simulink library "measurement_tools"  (Simulink 8.6)
settings: Solver=ode45  SolverMode=SingleTasking  StartTime=0.0  StopTime=10.0  RelTol=1e-3
values from neighbouring files (symbols this model uses):
  D = 'STP4'    [digital_communications_gui.m]
undefined symbols (not defined in the file or in its folder): DiscIntNeverNeededParam, get
libraries: dspsigops x3, dspsnks4 x2, dspvision x2, simulink_extras x1, dspswit3 x1, dspobslib x1, simulink x1
settings Model: MAModelExclusionFileProxy=C:\Users\user\Desktop\HAW\Digital Communication Systems\labs\Matlab\measurement_tools_exclusions.xml  Creator=Schoenen  LastModifiedBy=user

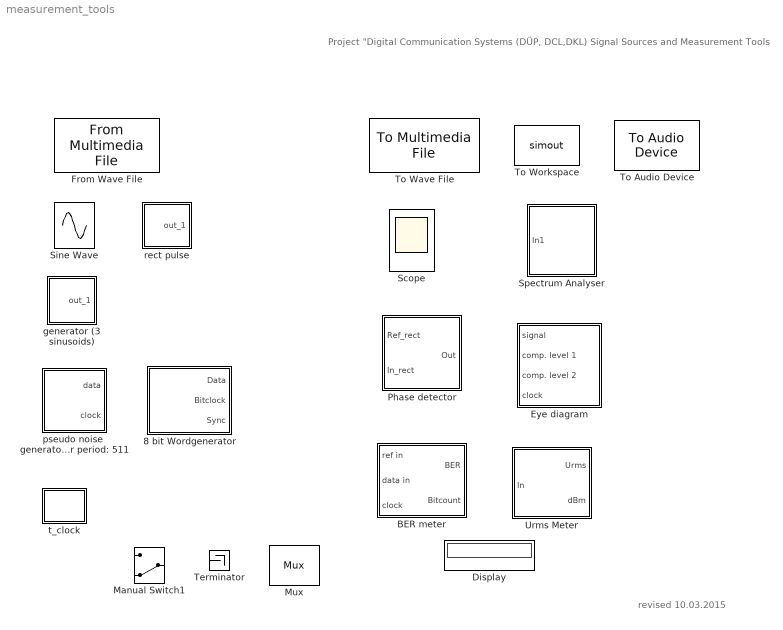
== system measurement_tools ==
  note: revised 10.03.2015
  note: Project "Digital Communication Systems (DÜP, DCL,DKL)
      | Signal Sources and Measurement Tools
  8 bit Wordgenerator : Subsystem  mask{word=[0 0 0 0 0 0 0 0], bt=1}
      mask prompts: word "8 Bit Word (enter vector)"; bt "Bitclock [Hz]"
      mask help: 8 Bit Wordgenerator
  BER meter : Subsystem
  Display : Display
      settings: Format=short_e
  Eye diagram : Subsystem  mask{Tsymb=1, Tfss=2/64e5, ns=4, ndisplay=1, ymin=1, ymax=1}
      mask prompts: Tsymb "symbol period [s]:"; Tfss "simulation step size [s]:"; ns "symbols per eye diagram (min. 4xndisplay):"; ndisplay "display time scale [ndisplay=number of symbols]:"
      mask init:
      | SampPerSymb = round(Tsymb/Tfss);
      | nsymb=ndisplay*ceil(ns/ndisplay);
  From Wave File : dspvision/From Multimedia File  inputFilename=audio_in_8kHz.wav  loop=on  numPlays=1  outputStreams=Audio only  videoDataType=single  audioDataType=double  inheritSampleTime=on  userDefinedSampleTime=1/30  noAudioOutput=off  isIntensityVideo=off  fourcc=RGB  colorVideoFormat=Separate color signals  outputEOF=off  dataOrg=Column-major  audioFrameSize=1  computeAudioFrameSize=off  outSamplingMode=Sample based
  Manual Switch1 : ManualSwitch  CurrentSetting=0
  Mux : Mux  Inputs=2
  Phase detector : Subsystem
  Scope : Scope
  Sine Wave : Sin  Amplitude=0  SampleTime=0
  Spectrum Analyser : Subsystem  mask{st=1}
      mask prompts: st "sample time [s]"
      mask help: Spectrum-Analyser
  Terminator : Terminator
  To Audio Device : dspsnks4/To Audio Device  deviceName=Default  inheritSampleRate=on  sampleRate=44100  deviceDatatype=Determine from input data type  autoBufferSize=on  bufferSize=4096  queueDuration=0.2  defaultOutputChannelMapping=on  outputChannelMapping=1:2  outputNumUnderrunSamples=off
  To Wave File : dspvision/To Multimedia File  outputFilename=audio_out.wav  streamSelection=Audio only  videoCompressor=None (uncompressed)  audioCompressor=None (uncompressed)  imagePorts=Separate color signals  fileType=WAV  audioDatatype=16-bit integer  fourcc=RGB  videoQuality=75  mj2000CompFactor=10
  To Workspace : ToWorkspace  VariableName=simout  SaveFormat=Structure  SampleTime=-1
  Urms Meter : Subsystem  mask{T=1}
      mask prompts: T "integration time [s]"
  generator (3 sinusoids) : Subsystem  mask(3_Tongenerator){}
      mask help: 3-Tongenerator
      mask init:
      | a1=@1(1); a2=@2(1); a3=@3(1); f1=@1(2); f2=@2(2); f3=@3(2); p1=@1(3); p2=@2(3); p3=@3(3);
      mask Help: Der Generator erzeugt eine Summe aus drei \nSinusschwingungen unterschiedlicher Amplitude \nund Phasenlage. Die Schwingungsparameter \nwerden jeweils als Vektor in der Form \n[Amplitude Frequenz Phase] eingegeben.
  pseudo noise  generator period: 511 : Subsystem  AncestorBlock=|  mask(pseudo noise generator){Tsymb=1, pol=unipolar, Tfss=2/64e5}
      | measuring_tools/pseudo noise
      |  generator
      | period: 511
      mask prompts: Tsymb "symbol period [s]"; pol "signal"; Tfss "simulation step size [s]"
      mask help: generates a periodical pseudo noise sequence (period Tp=511 Tbit)
      mask TypeOptions pol: bipolar | unipolar
  rect pulse : Subsystem  mask(Einheitsimpuls){breite=1, start=1}
      mask prompts: breite "width [s]"; start "start time [s]"
      mask help: Einheitsimpuls
      mask Help: Einheitsimpuls mit der Fläche 1
      mask Display: plot([0 0 0 0 1 0 0 0 0 0 0 0 0 0 0 0 0 0 0 0 ])
  t_clock : Subsystem
      mask init:
      | block_symbol=[0 1 0 0 0 0 0 0 0  1 0 0 0 0 0 0 01];
      mask Display: plot(block_symbol);

== system measurement_tools/8 bit Wordgenerator ==
  Clock-Generator : Subsystem  mask{bt=64e3}
      mask prompts: bt "Bitclock"
      mask help: Clock-Generator
  Parallel-Serial : Subsystem
  Word : Constant  Value=word
  Data : Outport
  Bitclock : Outport  Port=2
  Sync : Outport  Port=3
  wires:
  Parallel-Serial/1(Data_out) -> Data/1
  Word/1 -> Parallel-Serial/1(Data_in)
  Clock-Generator/2(Wordclock) -> Sync/1, Parallel-Serial/2(Preset)
  Clock-Generator/1(Bitclock) -> Bitclock/1, Parallel-Serial/3(Clock)

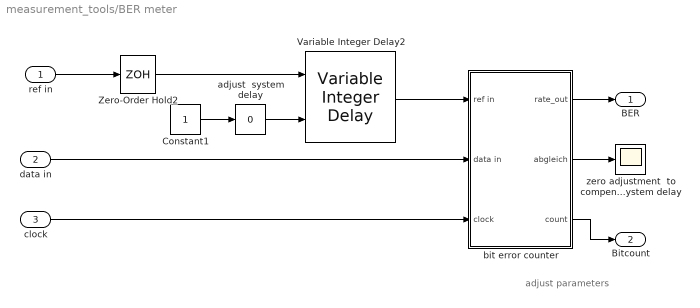
== system measurement_tools/BER meter ==
  note: adjust parameters
  ref in : Inport
  data in : Inport  Port=2
  clock : Inport  Port=3
  " bit error counter" : Subsystem  AncestorBlock=measuring_tools/discrete bit error counter  mask{Tbit=1, M=1}
      mask prompts: Tbit "bit period [s]"; M "measuring over number of bits:"
  Constant1 : Constant
  Variable Integer Delay2 : dspobslib/Variable Integer Delay  dmax=100  InputProcessing=Inherited (this choice will be removed - see release notes)  ic=0  noDFT=off
  Zero-Order Hold2 : ZeroOrderHold  SampleTime=2/64e5
  adjust  system delay : simulink/Math Operations/Slider Gain  low=0  gain=0  high=100
  zero adjustment  to compensate  system delay : Scope
  BER : Outport
  Bitcount : Outport  Port=2
  wires:
  " bit error counter"/3(count) -> Bitcount/1
  adjust  system delay/1 -> Variable Integer Delay2/2
  Constant1/1 -> adjust  system delay/1
  Zero-Order Hold2/1 -> Variable Integer Delay2/1
  Variable Integer Delay2/1 -> " bit error counter"/1(ref in)
  ref in/1 -> Zero-Order Hold2/1
  data in/1 -> " bit error counter"/2(data in)
  clock/1 -> " bit error counter"/3(clock)
  " bit error counter"/1(rate_out) -> BER/1
  " bit error counter"/2(abgleich) -> zero adjustment  to compensate  system delay/1

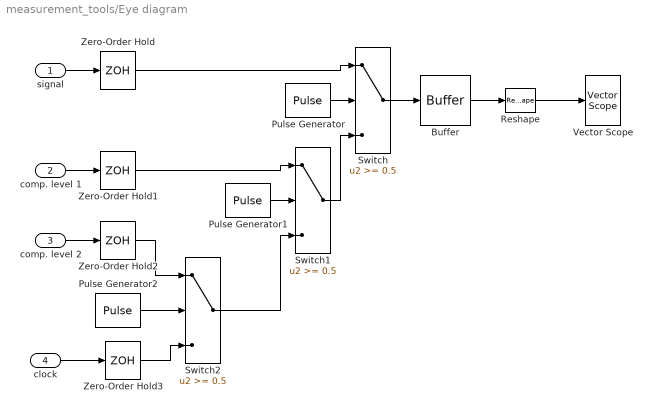
== system measurement_tools/Eye diagram ==
  signal : Inport
  comp. level 1 : Inport  Port=2
  comp. level 2 : Inport  Port=3
  clock : Inport  Port=4
  Buffer : Buffer  RequirementInfo="{}  %GIDa_20dddd1b_447a_4159_b5a4_549dd01b317e"  N=nsymb*SampPerSymb
  Pulse Generator : DiscretePulseGenerator  Period=nsymb*SampPerSymb  PulseWidth=(nsymb-3*ndisplay)*SampPerSymb  PhaseDelay=3*ndisplay*SampPerSymb  SampleTime=Tfss
  Pulse Generator1 : DiscretePulseGenerator  Period=nsymb*SampPerSymb  PulseWidth=ndisplay*SampPerSymb  SampleTime=Tfss
  Pulse Generator2 : DiscretePulseGenerator  Period=nsymb*SampPerSymb  PulseWidth=ndisplay*SampPerSymb  PhaseDelay=ndisplay*SampPerSymb  SampleTime=Tfss
  Reshape : Reshape  OutputDimensionality=Customize  OutputDimensions=[ndisplay*SampPerSymb,nsymb/ndisplay]
  Switch : Switch  Threshold=0.5  SaturateOnIntegerOverflow=on
  Switch1 : Switch  Threshold=0.5  SaturateOnIntegerOverflow=on
  Switch2 : Switch  Threshold=0.5  SaturateOnIntegerOverflow=on
  Vector Scope : dspsnks4/Vector Scope  ScopeProperties=off  Domain=Time  HorizSpan=1  DisplayProperties=off  AxisGrid=on  Memory=on  FrameNumber=on  AxisLegend=off  AxisZoom=off  OpenScopeAtSimStart=on  OpenScopeImmediately=off  FigPos=get(0,'defaultfigureposition')  AxisProperties=on  XUnits=Hertz  XRange=[0...Fs/2]  InheritXIncr=on  XIncr=1  XLabel=Time  XLimit=Auto  XMin=0  XMax=1  XStart=0  YUnits=dB  YLabel=Amplitude  LineProperties=off  LineColors=[1 0 0]|[0 1 0]|[0 0 1]  XAxisParamsVer=6.8
      settings: YMin=ymin  YMax=ymax
  Zero-Order Hold{,1..3} (4 alike) : ZeroOrderHold  SampleTime=Tfss
  wires:
  Pulse Generator2/1 -> Switch2/2
  Switch2/1 -> Switch1/3
  Zero-Order Hold3/1 -> Switch2/3
  clock/1 -> Zero-Order Hold3/1
  Zero-Order Hold2/1 -> Switch2/1
  comp. level 2/1 -> Zero-Order Hold2/1
  comp. level 1/1 -> Zero-Order Hold1/1
  signal/1 -> Zero-Order Hold/1
  Switch1/1 -> Switch/3
  Pulse Generator1/1 -> Switch1/2
  Zero-Order Hold1/1 -> Switch1/1
  Pulse Generator/1 -> Switch/2
  Switch/1 -> Buffer/1
  Zero-Order Hold/1 -> Switch/1
  Reshape/1 -> Vector Scope/1
  Buffer/1 -> Reshape/1

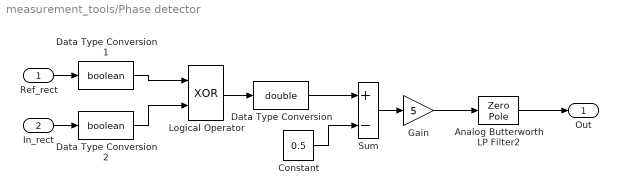
== system measurement_tools/Phase detector ==
  Ref_rect : Inport
  In_rect : Inport  Port=2
  Analog Butterworth LP Filter2 : ZeroPole  Zeros=z  Poles=p  Gain=k  mask(buttap){}
      mask help:
      | Analog Butterworth low pass filter.
      |
      | (Requires Signal Processing Toolbox)
      mask init:
      | [z,p,k]=buttap(@2); z=@1*z; p=@1*p; k=real(prod(-p)); [num,den]=zp2tf(z,p,k); w=logspace(log10(@1/10),log10(10*@1),20); h=freqs(num,den,w);
      mask Help: Butterworth low pass filter using MATLAB's butter command.
      mask Display: plot(20*log10(w),20*log10(abs(h)))
  Constant : Constant  Value=0.5
  Data Type Conversion : DataTypeConversion  OutDataTypeStr=double  SaturateOnIntegerOverflow=on  RndMeth=Zero
  Data Type Conversion1 : DataTypeConversion  OutDataTypeStr=boolean  SaturateOnIntegerOverflow=on  RndMeth=Zero
  Data Type Conversion2 : DataTypeConversion  OutDataTypeStr=boolean  SaturateOnIntegerOverflow=on  RndMeth=Zero
  Gain : Gain  Gain=5  SaturateOnIntegerOverflow=on  OutDataTypeStr=Inherit: Same as input  ParamDataTypeStr=Inherit: Same as input
  Logical Operator : Logic  Operator=XOR
  Sum : Sum  Inputs=+-  SaturateOnIntegerOverflow=on
  Out : Outport
  wires:
  In_rect/1 -> Data Type Conversion2/1
  Gain/1 -> Analog Butterworth LP Filter2/1
  Ref_rect/1 -> Data Type Conversion1/1
  Sum/1 -> Gain/1
  Constant/1 -> Sum/2
  Data Type Conversion/1 -> Sum/1
  Logical Operator/1 -> Data Type Conversion/1
  Data Type Conversion2/1 -> Logical Operator/2
  Data Type Conversion1/1 -> Logical Operator/1
  Analog Butterworth LP Filter2/1 -> Out/1

== system measurement_tools/Spectrum Analyser ==
  In1 : Inport
  Spectrum Scope : SpectrumAnalyzer
  Zero-Order Hold : ZeroOrderHold  SampleTime=st
  wires:
  In1/1 -> Zero-Order Hold/1
  Zero-Order Hold/1 -> Spectrum Scope/1

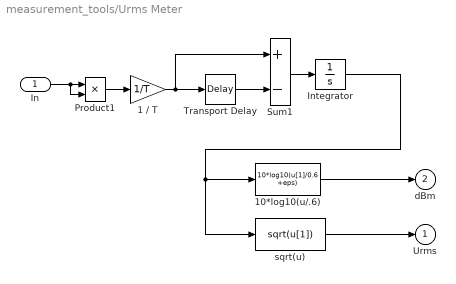
== system measurement_tools/Urms Meter ==
  In : Inport
  1 / T : Gain  Gain=1/T  SaturateOnIntegerOverflow=on  OutDataTypeStr=Inherit: Same as input  ParamDataTypeStr=Inherit: Same as input
  10*log10(u/.6) : Fcn  Expr=10*log10(u[1]/0.6 +eps)
  Integrator : Integrator
  Product1 : Product  SaturateOnIntegerOverflow=on  InputSameDT=on  OutDataTypeStr=Inherit: Same as first input
  Sum1 : Sum  Inputs=+-  SaturateOnIntegerOverflow=on  InputSameDT=on  OutDataTypeStr=Inherit: Same as first input
  Transport Delay : TransportDelay  DelayTime=T  BufferSize=1024*8
  sqrt(u) : Fcn  Expr=sqrt(u[1])
  Urms : Outport  InitialOutput=0
  dBm : Outport  Port=2  InitialOutput=0
  wires:
  sqrt(u)/1 -> Urms/1
  In/1 -> Product1/2, Product1/1
  Sum1/1 -> Integrator/1
  Transport Delay/1 -> Sum1/2
  1 / T/1 -> Sum1/1, Transport Delay/1
  Integrator/1 -> 10*log10(u/.6)/1, sqrt(u)/1
  10*log10(u/.6)/1 -> dBm/1
  Product1/1 -> 1 / T/1

== system measurement_tools/generator (3 sinusoids) ==
  Clock : Clock
  NF : Fcn  Expr=a1*sin(2*pi*f1*u+p1)
  NF1 : Fcn  Expr=a2*sin(2*pi*f2*u+p2)
  NF4 : Fcn  Expr=a3*sin(2*pi*f3*u+p3)
  Sum : Sum  Inputs=+++  SaturateOnIntegerOverflow=on  InputSameDT=on  OutDataTypeStr=Inherit: Same as first input
  out_1 : Outport
  wires:
  Sum/1 -> out_1/1
  NF/1 -> Sum/1
  NF1/1 -> Sum/2
  NF4/1 -> Sum/3
  Clock/1 -> NF1/1, NF/1, NF4/1

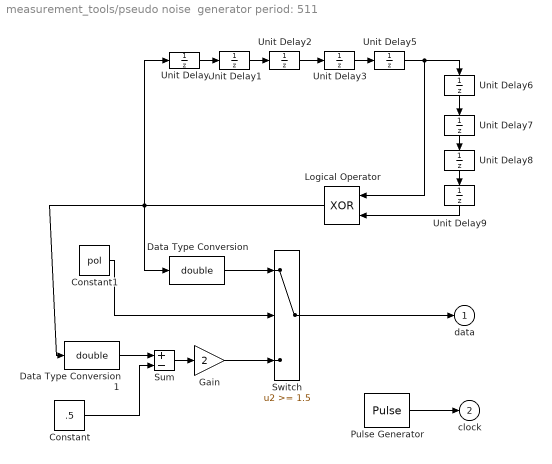
== system measurement_tools/pseudo noise  generator period: 511 ==
  Constant : Constant  Value=.5
  Constant1 : Constant  Value=pol
  Data Type Conversion : DataTypeConversion  OutDataTypeStr=double  SaturateOnIntegerOverflow=on  RndMeth=Zero
  Data Type Conversion1 : DataTypeConversion  OutDataTypeStr=double  SaturateOnIntegerOverflow=on  RndMeth=Zero
  Gain : Gain  Gain=2  SaturateOnIntegerOverflow=on  OutDataTypeStr=Inherit: Same as input  ParamDataTypeStr=Inherit: Same as input
  Logical Operator : Logic  Operator=XOR
  Pulse Generator : DiscretePulseGenerator  Period=round(Tsymb/Tfss)  SampleTime=Tfss
  Sum : Sum  Inputs=+-  SaturateOnIntegerOverflow=on  InputSameDT=on  OutDataTypeStr=Inherit: Same as first input
  Switch : Switch  Threshold=1.5  SaturateOnIntegerOverflow=on  InputSameDT=on
  Unit Delay : UnitDelay  InitialCondition=1  SampleTime=Tsymb
  Unit Delay{1..3,5..9} (8 alike) : UnitDelay  SampleTime=Tsymb
  data : Outport  InitialOutput=0
  clock : Outport  Port=2
  wires:
  Pulse Generator/1 -> clock/1
  Constant1/1 -> Switch/2
  Logical Operator/1 -> Unit Delay/1, Data Type Conversion1/1, Data Type Conversion/1
  Gain/1 -> Switch/3
  Switch/1 -> data/1
  Constant/1 -> Sum/2
  Sum/1 -> Gain/1
  Unit Delay5/1 -> Unit Delay6/1, Logical Operator/1
  Unit Delay3/1 -> Unit Delay5/1
  Unit Delay2/1 -> Unit Delay3/1
  Unit Delay9/1 -> Logical Operator/2
  Unit Delay8/1 -> Unit Delay9/1
  Unit Delay7/1 -> Unit Delay8/1
  Unit Delay6/1 -> Unit Delay7/1
  Unit Delay/1 -> Unit Delay1/1
  Unit Delay1/1 -> Unit Delay2/1
  Data Type Conversion1/1 -> Sum/1
  Data Type Conversion/1 -> Switch/1

== system measurement_tools/rect pulse ==
  Step Input : Step  Time=start  After=1/breite  SampleTime=breite
  Sum : Sum  Inputs=+-  SaturateOnIntegerOverflow=on  InputSameDT=on  OutDataTypeStr=Inherit: Same as first input
  Unit Delay : UnitDelay  SampleTime=breite
  out_1 : Outport
  wires:
  Sum/1 -> out_1/1
  Unit Delay/1 -> Sum/2
  Step Input/1 -> Unit Delay/1, Sum/1

== system measurement_tools/t_clock ==
  Clock : Clock
  To Workspace : ToWorkspace  VariableName=t_clock  SampleTime=0.5/64e3
      settings: MaxDataPoints=10000
  wires:
  Clock/1 -> To Workspace/1

== system measurement_tools/8 bit Wordgenerator/Clock-Generator ==
  Clock : simulink_extras/Flip Flops/Clock  period=1/bt
  Constant1 : Constant  Value=7
  Counter : dspswit3/Counter  Direction=Up  CountEvent=Rising edge  CounterSize=User defined  MaxCount=7  InitialCount=0  Output=Count  HitValue=32  ResetInput=off  SamplesPerFrame=1  Ts=1  CntDtype=double  HitDtype=Logical
  Relational Operator : RelationalOperator  Operator===
  Bitclock : Outport
  Wordclock : Outport  Port=2
  wires:
  Relational Operator/1 -> Wordclock/1
  Constant1/1 -> Relational Operator/2
  Counter/1 -> Relational Operator/1
  Clock/1 -> Bitclock/1, Counter/1

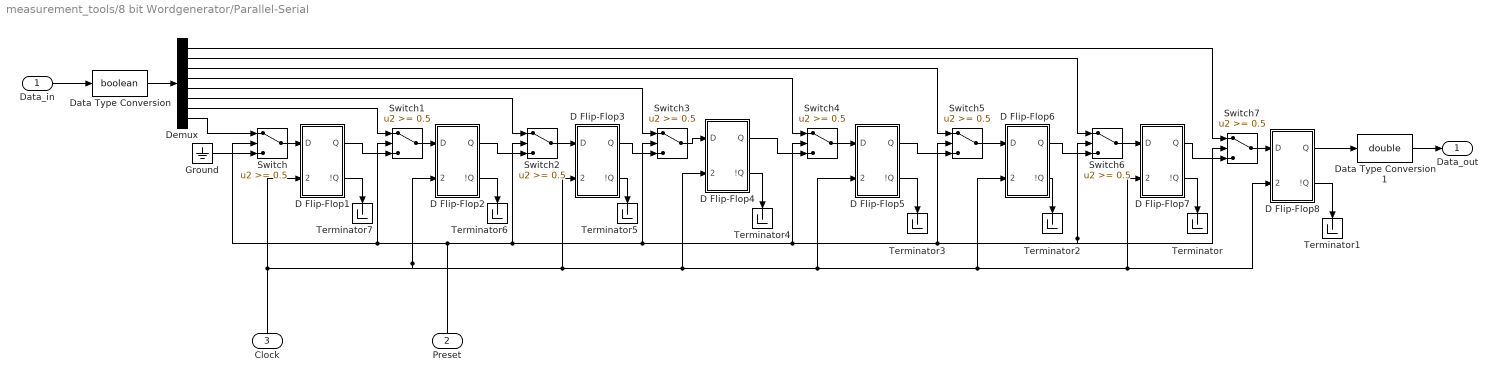
== system measurement_tools/8 bit Wordgenerator/Parallel-Serial ==
  Data_in : Inport
  Preset : Inport  Port=2
  Clock : Inport  Port=3
  D Flip-Flop1 : Subsystem  AncestorBlock=simulink_extras/Flip Flops/D Flip-Flop  mask(DFlipFlop){}
      mask help: D Flip-Flop Block
      mask Help:
      | The D flip-flop block has the following characteristic table:
      | <pre>
      |   Q(t)  D(t)     Q(tnext)
      |   ------------------------
      |    0      0       0
      |    0      1       1
      |    1      0       0
      |    1      1       1
      | </pre>
      | Q(tnext) refers to the output on a clock pulse (CLK) rising edge and when the
      | chip is enabled (!CLR ~= 0).
      | <br><br>
      | The D flip-flop transfers "data" into a memory element (flip-flop) on each clock
      | pulse (CLK). The chip enable input signal, !CLR, is sometimes given the
      | designation G (for gate) to indicate that this input enables the gated latch
      | allowing data entry into the flip-flop.
  D Flip-Flop2 : Subsystem  AncestorBlock=simulink_extras/Flip Flops/D Flip-Flop  mask(DFlipFlop){}
      mask help: D Flip-Flop Block
      mask Help:
      | The D flip-flop block has the following characteristic table:
      | <pre>
      |   Q(t)  D(t)     Q(tnext)
      |   ------------------------
      |    0      0       0
      |    0      1       1
      |    1      0       0
      |    1      1       1
      | </pre>
      | Q(tnext) refers to the output on a clock pulse (CLK) rising edge and when the
      | chip is enabled (!CLR ~= 0).
      | <br><br>
      | The D flip-flop transfers "data" into a memory element (flip-flop) on each clock
      | pulse (CLK). The chip enable input signal, !CLR, is sometimes given the
      | designation G (for gate) to indicate that this input enables the gated latch
      | allowing data entry into the flip-flop.
  D Flip-Flop3 : Subsystem  AncestorBlock=simulink_extras/Flip Flops/D Flip-Flop  mask(DFlipFlop){}
      mask help: D Flip-Flop Block
      mask Help:
      | The D flip-flop block has the following characteristic table:
      | <pre>
      |   Q(t)  D(t)     Q(tnext)
      |   ------------------------
      |    0      0       0
      |    0      1       1
      |    1      0       0
      |    1      1       1
      | </pre>
      | Q(tnext) refers to the output on a clock pulse (CLK) rising edge and when the
      | chip is enabled (!CLR ~= 0).
      | <br><br>
      | The D flip-flop transfers "data" into a memory element (flip-flop) on each clock
      | pulse (CLK). The chip enable input signal, !CLR, is sometimes given the
      | designation G (for gate) to indicate that this input enables the gated latch
      | allowing data entry into the flip-flop.
  D Flip-Flop4 : Subsystem  AncestorBlock=simulink_extras/Flip Flops/D Flip-Flop  mask(DFlipFlop){}
      mask help: D Flip-Flop Block
      mask Help:
      | The D flip-flop block has the following characteristic table:
      | <pre>
      |   Q(t)  D(t)     Q(tnext)
      |   ------------------------
      |    0      0       0
      |    0      1       1
      |    1      0       0
      |    1      1       1
      | </pre>
      | Q(tnext) refers to the output on a clock pulse (CLK) rising edge and when the
      | chip is enabled (!CLR ~= 0).
      | <br><br>
      | The D flip-flop transfers "data" into a memory element (flip-flop) on each clock
      | pulse (CLK). The chip enable input signal, !CLR, is sometimes given the
      | designation G (for gate) to indicate that this input enables the gated latch
      | allowing data entry into the flip-flop.
  D Flip-Flop5 : Subsystem  AncestorBlock=simulink_extras/Flip Flops/D Flip-Flop  mask(DFlipFlop){}
      mask help: D Flip-Flop Block
      mask Help:
      | The D flip-flop block has the following characteristic table:
      | <pre>
      |   Q(t)  D(t)     Q(tnext)
      |   ------------------------
      |    0      0       0
      |    0      1       1
      |    1      0       0
      |    1      1       1
      | </pre>
      | Q(tnext) refers to the output on a clock pulse (CLK) rising edge and when the
      | chip is enabled (!CLR ~= 0).
      | <br><br>
      | The D flip-flop transfers "data" into a memory element (flip-flop) on each clock
      | pulse (CLK). The chip enable input signal, !CLR, is sometimes given the
      | designation G (for gate) to indicate that this input enables the gated latch
      | allowing data entry into the flip-flop.
  D Flip-Flop6 : Subsystem  AncestorBlock=simulink_extras/Flip Flops/D Flip-Flop  mask(DFlipFlop){}
      mask help: D Flip-Flop Block
      mask Help:
      | The D flip-flop block has the following characteristic table:
      | <pre>
      |   Q(t)  D(t)     Q(tnext)
      |   ------------------------
      |    0      0       0
      |    0      1       1
      |    1      0       0
      |    1      1       1
      | </pre>
      | Q(tnext) refers to the output on a clock pulse (CLK) rising edge and when the
      | chip is enabled (!CLR ~= 0).
      | <br><br>
      | The D flip-flop transfers "data" into a memory element (flip-flop) on each clock
      | pulse (CLK). The chip enable input signal, !CLR, is sometimes given the
      | designation G (for gate) to indicate that this input enables the gated latch
      | allowing data entry into the flip-flop.
  D Flip-Flop7 : Subsystem  AncestorBlock=simulink_extras/Flip Flops/D Flip-Flop  mask(DFlipFlop){}
      mask help: D Flip-Flop Block
      mask Help:
      | The D flip-flop block has the following characteristic table:
      | <pre>
      |   Q(t)  D(t)     Q(tnext)
      |   ------------------------
      |    0      0       0
      |    0      1       1
      |    1      0       0
      |    1      1       1
      | </pre>
      | Q(tnext) refers to the output on a clock pulse (CLK) rising edge and when the
      | chip is enabled (!CLR ~= 0).
      | <br><br>
      | The D flip-flop transfers "data" into a memory element (flip-flop) on each clock
      | pulse (CLK). The chip enable input signal, !CLR, is sometimes given the
      | designation G (for gate) to indicate that this input enables the gated latch
      | allowing data entry into the flip-flop.
  D Flip-Flop8 : Subsystem  AncestorBlock=simulink_extras/Flip Flops/D Flip-Flop  mask(DFlipFlop){}
      mask help: D Flip-Flop Block
      mask Help:
      | The D flip-flop block has the following characteristic table:
      | <pre>
      |   Q(t)  D(t)     Q(tnext)
      |   ------------------------
      |    0      0       0
      |    0      1       1
      |    1      0       0
      |    1      1       1
      | </pre>
      | Q(tnext) refers to the output on a clock pulse (CLK) rising edge and when the
      | chip is enabled (!CLR ~= 0).
      | <br><br>
      | The D flip-flop transfers "data" into a memory element (flip-flop) on each clock
      | pulse (CLK). The chip enable input signal, !CLR, is sometimes given the
      | designation G (for gate) to indicate that this input enables the gated latch
      | allowing data entry into the flip-flop.
  Data Type Conversion : DataTypeConversion  OutDataTypeStr=boolean  SaturateOnIntegerOverflow=on  RndMeth=Zero
  Data Type Conversion1 : DataTypeConversion  OutDataTypeStr=double  SaturateOnIntegerOverflow=on  RndMeth=Zero
  Demux : Demux  Outputs=8
  Ground : Ground
  Switch{,1..7} (8 alike) : Switch  Threshold=0.5  SaturateOnIntegerOverflow=on
  Terminator{,1..7} (8 alike) : Terminator
  Data_out : Outport
  wires:
  Data Type Conversion1/1 -> Data_out/1
  D Flip-Flop8/1(Q) -> Data Type Conversion1/1
  Preset/1 -> Switch7/2, Switch6/2, Switch5/2, Switch4/2, Switch3/2, Switch2/2, Switch1/2, Switch/2
  Clock/1 -> D Flip-Flop1/2(CLK), D Flip-Flop2/2(CLK), D Flip-Flop3/2(CLK), D Flip-Flop4/2(CLK), D Flip-Flop5/2(CLK), D Flip-Flop6/2(CLK), D Flip-Flop8/2(CLK), D Flip-Flop7/2(CLK)
  Data_in/1 -> Data Type Conversion/1
  Data Type Conversion/1 -> Demux/1
  D Flip-Flop1/2(!Q) -> Terminator7/1
  D Flip-Flop2/2(!Q) -> Terminator6/1
  D Flip-Flop3/2(!Q) -> Terminator5/1
  D Flip-Flop4/2(!Q) -> Terminator4/1
  D Flip-Flop5/2(!Q) -> Terminator3/1
  D Flip-Flop6/2(!Q) -> Terminator2/1
  D Flip-Flop8/2(!Q) -> Terminator1/1
  D Flip-Flop7/2(!Q) -> Terminator/1
  Demux/1 -> Switch7/1
  Demux/2 -> Switch6/1
  Demux/3 -> Switch5/1
  Demux/4 -> Switch4/1
  Demux/5 -> Switch3/1
  Demux/6 -> Switch2/1
  Demux/7 -> Switch1/1
  Demux/8 -> Switch/1
  D Flip-Flop3/1(Q) -> Switch3/3
  D Flip-Flop7/1(Q) -> Switch7/3
  D Flip-Flop5/1(Q) -> Switch5/3
  Switch7/1 -> D Flip-Flop8/1(D)
  D Flip-Flop6/1(Q) -> Switch6/3
  Switch6/1 -> D Flip-Flop7/1(D)
  Switch5/1 -> D Flip-Flop6/1(D)
  D Flip-Flop4/1(Q) -> Switch4/3
  Switch4/1 -> D Flip-Flop5/1(D)
  Switch3/1 -> D Flip-Flop4/1(D)
  D Flip-Flop2/1(Q) -> Switch2/3
  Switch2/1 -> D Flip-Flop3/1(D)
  Ground/1 -> Switch/3
  D Flip-Flop1/1(Q) -> Switch1/3
  Switch1/1 -> D Flip-Flop2/1(D)
  Switch/1 -> D Flip-Flop1/1(D)

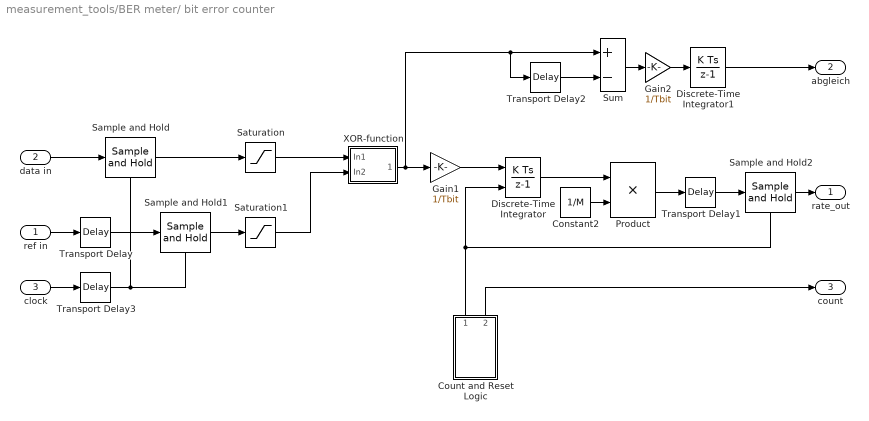
== system measurement_tools/BER meter/ bit error counter ==
  ref in : Inport
  data in : Inport  Port=2
  clock : Inport  Port=3
  Constant2 : Constant  Value=1/M
  Count and Reset Logic : Subsystem
  Discrete-Time Integrator : DiscreteIntegrator  ExternalReset=level  SampleTime=Tbit  ICPrevOutput=DiscIntNeverNeededParam  ICPrevScaledInput=DiscIntNeverNeededParam
  Discrete-Time Integrator1 : DiscreteIntegrator  SampleTime=Tbit  ICPrevOutput=DiscIntNeverNeededParam  ICPrevScaledInput=DiscIntNeverNeededParam
  Gain1 : Gain  Gain=1/Tbit  SaturateOnIntegerOverflow=on  OutDataTypeStr=Inherit: Same as input  ParamDataTypeStr=Inherit: Same as input
  Gain2 : Gain  Gain=1/Tbit  SaturateOnIntegerOverflow=on  OutDataTypeStr=Inherit: Same as input  ParamDataTypeStr=Inherit: Same as input
  Product : Product  SaturateOnIntegerOverflow=on  OutDataTypeStr=Inherit: Same as first input
  Sample and Hold : dspsigops/Sample and Hold  trig=Rising edge  initCond=0  latchinput=off
  Sample and Hold1 : dspsigops/Sample and Hold  trig=Rising edge  initCond=0  latchinput=off
  Sample and Hold2 : dspsigops/Sample and Hold  trig=Rising edge  initCond=0  latchinput=off
  Saturation : Saturate  UpperLimit=1  LowerLimit=0
  Saturation1 : Saturate  UpperLimit=1  LowerLimit=0
  Sum : Sum  Inputs=+-  SaturateOnIntegerOverflow=on
  Transport Delay : TransportDelay  DelayTime=0.5*Tbit
  Transport Delay1 : TransportDelay  DelayTime=0.5*Tbit
  Transport Delay2 : TransportDelay  DelayTime=15*Tbit
  Transport Delay3 : TransportDelay  DelayTime=0.5*Tbit
  XOR-function : Subsystem
  rate_out : Outport  InitialOutput=0
  abgleich : Outport  Port=2  InitialOutput=0
  count : Outport  Port=3  InitialOutput=0
  wires:
  Count and Reset Logic/2(count) -> count/1
  Transport Delay/1 -> Sample and Hold1/1
  Transport Delay1/1 -> Sample and Hold2/1
  Constant2/1 -> Product/2
  Sample and Hold2/1 -> rate_out/1
  Product/1 -> Transport Delay1/1
  Discrete-Time Integrator/1 -> Product/1
  Gain1/1 -> Discrete-Time Integrator/1
  Count and Reset Logic/1(reset) -> Sample and Hold2/Trigger, Discrete-Time Integrator/2
  Sample and Hold1/1 -> Saturation1/1
  Transport Delay3/1 -> Sample and Hold1/Trigger, Sample and Hold/Trigger
  clock/1 -> Transport Delay3/1
  Sample and Hold/1 -> Saturation/1
  Saturation1/1 -> XOR-function/2(In2)
  ref in/1 -> Transport Delay/1
  Saturation/1 -> XOR-function/1(In1)
  data in/1 -> Sample and Hold/1
  XOR-function/1(Out1) -> Sum/1, Transport Delay2/1, Gain1/1
  Transport Delay2/1 -> Sum/2
  Sum/1 -> Gain2/1
  Discrete-Time Integrator1/1 -> abgleich/1
  Gain2/1 -> Discrete-Time Integrator1/1

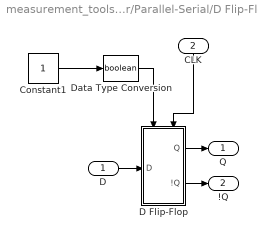
== system measurement_tools/8 bit Wordgenerator/Parallel-Serial/D Flip-Flop1 ==
  D : Inport
  CLK : Inport  Port=2
  Constant1 : Constant
  D Flip-Flop : Subsystem  TreatAsAtomicUnit=on
  Data Type Conversion : DataTypeConversion  OutDataTypeStr=boolean  SaturateOnIntegerOverflow=on  RndMeth=Zero
  Q : Outport  InitialOutput=0
  !Q : Outport  Port=2  InitialOutput=1
  wires:
  Constant1/1 -> Data Type Conversion/1
  Data Type Conversion/1 -> D Flip-Flop/Enable
  CLK/1 -> D Flip-Flop/Trigger
  D Flip-Flop/1(Q) -> Q/1
  D/1 -> D Flip-Flop/1(D)
  D Flip-Flop/2(!Q) -> !Q/1

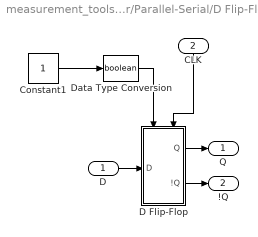
== system measurement_tools/8 bit Wordgenerator/Parallel-Serial/D Flip-Flop2 ==
  D : Inport
  CLK : Inport  Port=2
  Constant1 : Constant
  D Flip-Flop : Subsystem  TreatAsAtomicUnit=on
  Data Type Conversion : DataTypeConversion  OutDataTypeStr=boolean  SaturateOnIntegerOverflow=on  RndMeth=Zero
  Q : Outport  InitialOutput=0
  !Q : Outport  Port=2  InitialOutput=1
  wires:
  Constant1/1 -> Data Type Conversion/1
  Data Type Conversion/1 -> D Flip-Flop/Enable
  CLK/1 -> D Flip-Flop/Trigger
  D Flip-Flop/1(Q) -> Q/1
  D/1 -> D Flip-Flop/1(D)
  D Flip-Flop/2(!Q) -> !Q/1

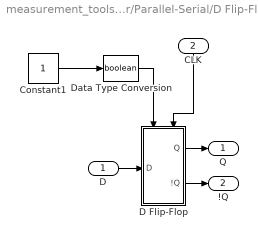
== system measurement_tools/8 bit Wordgenerator/Parallel-Serial/D Flip-Flop3 ==
  D : Inport
  CLK : Inport  Port=2
  Constant1 : Constant
  D Flip-Flop : Subsystem  TreatAsAtomicUnit=on
  Data Type Conversion : DataTypeConversion  OutDataTypeStr=boolean  SaturateOnIntegerOverflow=on  RndMeth=Zero
  Q : Outport  InitialOutput=0
  !Q : Outport  Port=2  InitialOutput=1
  wires:
  Constant1/1 -> Data Type Conversion/1
  Data Type Conversion/1 -> D Flip-Flop/Enable
  CLK/1 -> D Flip-Flop/Trigger
  D Flip-Flop/1(Q) -> Q/1
  D/1 -> D Flip-Flop/1(D)
  D Flip-Flop/2(!Q) -> !Q/1

== system measurement_tools/8 bit Wordgenerator/Parallel-Serial/D Flip-Flop4 ==
  D : Inport
  CLK : Inport  Port=2
  Constant1 : Constant
  D Flip-Flop : Subsystem  TreatAsAtomicUnit=on
  Data Type Conversion : DataTypeConversion  OutDataTypeStr=boolean  SaturateOnIntegerOverflow=on  RndMeth=Zero
  Q : Outport  InitialOutput=0
  !Q : Outport  Port=2  InitialOutput=1
  wires:
  Constant1/1 -> Data Type Conversion/1
  Data Type Conversion/1 -> D Flip-Flop/Enable
  CLK/1 -> D Flip-Flop/Trigger
  D Flip-Flop/1(Q) -> Q/1
  D/1 -> D Flip-Flop/1(D)
  D Flip-Flop/2(!Q) -> !Q/1

== system measurement_tools/8 bit Wordgenerator/Parallel-Serial/D Flip-Flop5 ==
  D : Inport
  CLK : Inport  Port=2
  Constant1 : Constant
  D Flip-Flop : Subsystem  TreatAsAtomicUnit=on
  Data Type Conversion : DataTypeConversion  OutDataTypeStr=boolean  SaturateOnIntegerOverflow=on  RndMeth=Zero
  Q : Outport  InitialOutput=0
  !Q : Outport  Port=2  InitialOutput=1
  wires:
  Constant1/1 -> Data Type Conversion/1
  Data Type Conversion/1 -> D Flip-Flop/Enable
  CLK/1 -> D Flip-Flop/Trigger
  D Flip-Flop/1(Q) -> Q/1
  D/1 -> D Flip-Flop/1(D)
  D Flip-Flop/2(!Q) -> !Q/1

== system measurement_tools/8 bit Wordgenerator/Parallel-Serial/D Flip-Flop6 ==
  D : Inport
  CLK : Inport  Port=2
  Constant1 : Constant
  D Flip-Flop : Subsystem  TreatAsAtomicUnit=on
  Data Type Conversion : DataTypeConversion  OutDataTypeStr=boolean  SaturateOnIntegerOverflow=on  RndMeth=Zero
  Q : Outport  InitialOutput=0
  !Q : Outport  Port=2  InitialOutput=1
  wires:
  Constant1/1 -> Data Type Conversion/1
  Data Type Conversion/1 -> D Flip-Flop/Enable
  CLK/1 -> D Flip-Flop/Trigger
  D Flip-Flop/1(Q) -> Q/1
  D/1 -> D Flip-Flop/1(D)
  D Flip-Flop/2(!Q) -> !Q/1

== system measurement_tools/8 bit Wordgenerator/Parallel-Serial/D Flip-Flop7 ==
  D : Inport
  CLK : Inport  Port=2
  Constant1 : Constant
  D Flip-Flop : Subsystem  TreatAsAtomicUnit=on
  Data Type Conversion : DataTypeConversion  OutDataTypeStr=boolean  SaturateOnIntegerOverflow=on  RndMeth=Zero
  Q : Outport  InitialOutput=0
  !Q : Outport  Port=2  InitialOutput=1
  wires:
  Constant1/1 -> Data Type Conversion/1
  Data Type Conversion/1 -> D Flip-Flop/Enable
  CLK/1 -> D Flip-Flop/Trigger
  D Flip-Flop/1(Q) -> Q/1
  D/1 -> D Flip-Flop/1(D)
  D Flip-Flop/2(!Q) -> !Q/1

== system measurement_tools/8 bit Wordgenerator/Parallel-Serial/D Flip-Flop8 ==
  D : Inport
  CLK : Inport  Port=2
  Constant1 : Constant
  D Flip-Flop : Subsystem  TreatAsAtomicUnit=on
  Data Type Conversion : DataTypeConversion  OutDataTypeStr=boolean  SaturateOnIntegerOverflow=on  RndMeth=Zero
  Q : Outport  InitialOutput=0
  !Q : Outport  Port=2  InitialOutput=1
  wires:
  Constant1/1 -> Data Type Conversion/1
  Data Type Conversion/1 -> D Flip-Flop/Enable
  CLK/1 -> D Flip-Flop/Trigger
  D Flip-Flop/1(Q) -> Q/1
  D/1 -> D Flip-Flop/1(D)
  D Flip-Flop/2(!Q) -> !Q/1

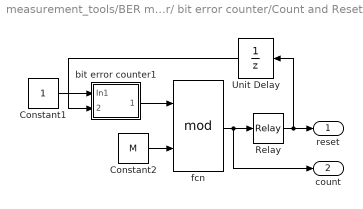
== system measurement_tools/BER meter/ bit error counter/Count and Reset Logic ==
  Constant1 : Constant
  Constant2 : Constant  Value=M
  Relay : Relay  OnSwitchValue=M-1.5  OffSwitchValue=M-1.5
  Unit Delay : UnitDelay  SampleTime=Tbit
  bit error counter1 : Subsystem
  fcn : Math  Operator=mod  SaturateOnIntegerOverflow=on
  reset : Outport
  count : Outport  Port=2
  wires:
  Unit Delay/1 -> bit error counter1/2(reset)
  Relay/1 -> Unit Delay/1, reset/1
  fcn/1 -> count/1, Relay/1
  Constant1/1 -> bit error counter1/1(In1)
  bit error counter1/1(Out1) -> fcn/1
  Constant2/1 -> fcn/2

== system measurement_tools/BER meter/ bit error counter/XOR-function ==
  In1 : Inport
  In2 : Inport  Port=2
  Constant : Constant  Value=2
  Math Function : Math  Operator=mod  SaturateOnIntegerOverflow=on
  Sum : Sum  SaturateOnIntegerOverflow=on  InputSameDT=on  OutDataTypeStr=Inherit: Same as first input
  Out1 : Outport  InitialOutput=0
  wires:
  Math Function/1 -> Out1/1
  Constant/1 -> Math Function/2
  Sum/1 -> Math Function/1
  In2/1 -> Sum/2
  In1/1 -> Sum/1

== system measurement_tools/8 bit Wordgenerator/Parallel-Serial/D Flip-Flop1/D Flip-Flop ==
  D : Inport  LatchByDelayingOutsideSignal=on
  C : EnablePort
  Trigger : TriggerPort
  Logic : Logic  Operator=NOT  Inputs=1
  Q : Outport  OutputWhenDisabled=reset  InitialOutput=0
  !Q : Outport  Port=2  OutputWhenDisabled=reset  InitialOutput=1
  wires:
  Logic/1 -> !Q/1
  D/1 -> Q/1, Logic/1

== system measurement_tools/8 bit Wordgenerator/Parallel-Serial/D Flip-Flop2/D Flip-Flop ==
  D : Inport  LatchByDelayingOutsideSignal=on
  C : EnablePort
  Trigger : TriggerPort
  Logic : Logic  Operator=NOT  Inputs=1
  Q : Outport  OutputWhenDisabled=reset  InitialOutput=0
  !Q : Outport  Port=2  OutputWhenDisabled=reset  InitialOutput=1
  wires:
  Logic/1 -> !Q/1
  D/1 -> Q/1, Logic/1

== system measurement_tools/8 bit Wordgenerator/Parallel-Serial/D Flip-Flop3/D Flip-Flop ==
  D : Inport  LatchByDelayingOutsideSignal=on
  C : EnablePort
  Trigger : TriggerPort
  Logic : Logic  Operator=NOT  Inputs=1
  Q : Outport  OutputWhenDisabled=reset  InitialOutput=0
  !Q : Outport  Port=2  OutputWhenDisabled=reset  InitialOutput=1
  wires:
  Logic/1 -> !Q/1
  D/1 -> Q/1, Logic/1

== system measurement_tools/8 bit Wordgenerator/Parallel-Serial/D Flip-Flop4/D Flip-Flop ==
  D : Inport  LatchByDelayingOutsideSignal=on
  C : EnablePort
  Trigger : TriggerPort
  Logic : Logic  Operator=NOT  Inputs=1
  Q : Outport  OutputWhenDisabled=reset  InitialOutput=0
  !Q : Outport  Port=2  OutputWhenDisabled=reset  InitialOutput=1
  wires:
  Logic/1 -> !Q/1
  D/1 -> Q/1, Logic/1

== system measurement_tools/8 bit Wordgenerator/Parallel-Serial/D Flip-Flop5/D Flip-Flop ==
  D : Inport  LatchByDelayingOutsideSignal=on
  C : EnablePort
  Trigger : TriggerPort
  Logic : Logic  Operator=NOT  Inputs=1
  Q : Outport  OutputWhenDisabled=reset  InitialOutput=0
  !Q : Outport  Port=2  OutputWhenDisabled=reset  InitialOutput=1
  wires:
  Logic/1 -> !Q/1
  D/1 -> Q/1, Logic/1

== system measurement_tools/8 bit Wordgenerator/Parallel-Serial/D Flip-Flop6/D Flip-Flop ==
  D : Inport  LatchByDelayingOutsideSignal=on
  C : EnablePort
  Trigger : TriggerPort
  Logic : Logic  Operator=NOT  Inputs=1
  Q : Outport  OutputWhenDisabled=reset  InitialOutput=0
  !Q : Outport  Port=2  OutputWhenDisabled=reset  InitialOutput=1
  wires:
  Logic/1 -> !Q/1
  D/1 -> Q/1, Logic/1

== system measurement_tools/8 bit Wordgenerator/Parallel-Serial/D Flip-Flop7/D Flip-Flop ==
  D : Inport  LatchByDelayingOutsideSignal=on
  C : EnablePort
  Trigger : TriggerPort
  Logic : Logic  Operator=NOT  Inputs=1
  Q : Outport  OutputWhenDisabled=reset  InitialOutput=0
  !Q : Outport  Port=2  OutputWhenDisabled=reset  InitialOutput=1
  wires:
  Logic/1 -> !Q/1
  D/1 -> Q/1, Logic/1

== system measurement_tools/8 bit Wordgenerator/Parallel-Serial/D Flip-Flop8/D Flip-Flop ==
  D : Inport  LatchByDelayingOutsideSignal=on
  C : EnablePort
  Trigger : TriggerPort
  Logic : Logic  Operator=NOT  Inputs=1
  Q : Outport  OutputWhenDisabled=reset  InitialOutput=0
  !Q : Outport  Port=2  OutputWhenDisabled=reset  InitialOutput=1
  wires:
  Logic/1 -> !Q/1
  D/1 -> Q/1, Logic/1

== system measurement_tools/BER meter/ bit error counter/Count and Reset Logic/bit error counter1 ==
  In1 : Inport
  reset : Inport  Port=2
  Constant1 : Constant  Value=0
  Sum : Sum  SaturateOnIntegerOverflow=on  InputSameDT=on  OutDataTypeStr=Inherit: Same as first input
  Switch : Switch  Threshold=0.5  SaturateOnIntegerOverflow=on
  Unit Delay : UnitDelay  SampleTime=Tbit
  Out1 : Outport  InitialOutput=0
  wires:
  reset/1 -> Switch/2
  Constant1/1 -> Switch/1
  Switch/1 -> Sum/2
  In1/1 -> Sum/1
  Unit Delay/1 -> Switch/3, Out1/1
  Sum/1 -> Unit Delay/1
